simulink library "fluidDynamicSurface_cl"  (R2018b)
settings: Solver=VariableStepAuto  StartTime=0.0  StopTime=10.0  RelTol=1e-3
undefined symbols (not defined in the file or in its folder): aeroStruct
libraries: vrlib x2, vectorNormalizer_ul x2, dynamicPressure_ul x1, alphaBeta_ul x1, surfaceCoefficients_ul x1
settings Model: Creator=mcobb  LastModifiedBy=mcobb

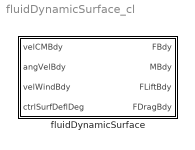
== system fluidDynamicSurface_cl ==
  fluidDynamicSurface : Subsystem  mask{aeroStruct=aeroStruct}
      mask prompts: aeroStruct "Aerodynamic surface structure"
      mask help:
      | Input must be an 1×N struct array with fields:
      |     refArea
      |     aeroCentPosVec
      |     spanUnitVec
      |     chordUnitVec
      |     fluidDensity
      |     CL
      |     CD
      |     alpha
      |     GainCL
      |     GainCD
      |
      | where N is the number of aerodynamic surfaces
      mask init:
      | fluidDynamicSurface_init

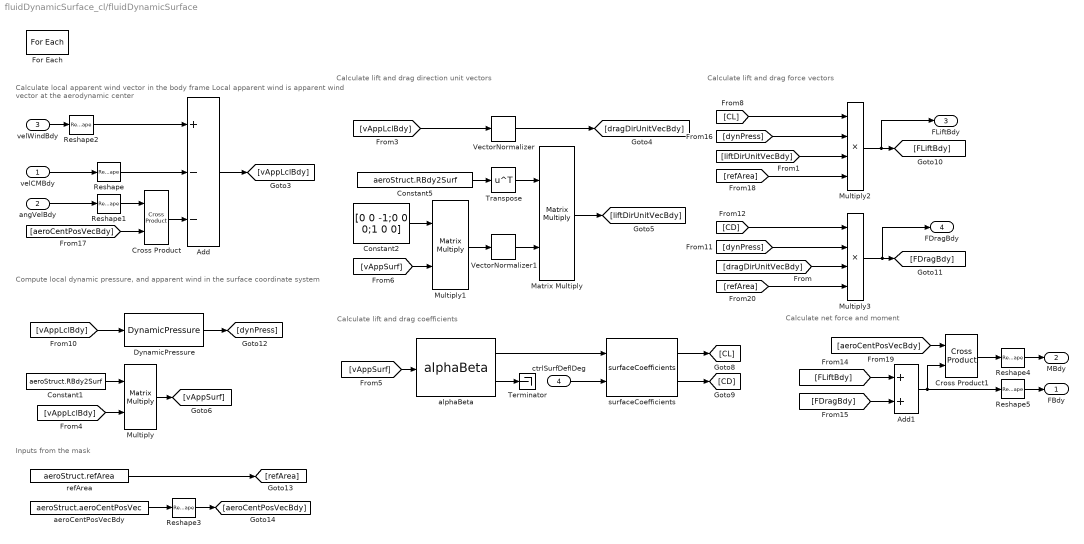
== system fluidDynamicSurface_cl/fluidDynamicSurface ==
  note: Calculate net force and moment
  note: Calculate lift and drag force vectors
  note: Calculate lift and drag coefficients
  note: Compute local dynamic pressure,
      | and apparent wind in the surface coordinate system
  note: Inputs from the mask
  note: Calculate lift and drag direction unit vectors
  note: Calculate local apparent wind vector in the body frame
      | Local apparent wind is apparent wind vector at the aerodynamic center
  velCMBdy : Inport
  angVelBdy : Inport  Port=2
  velWindBdy : Inport  Port=3
  ctrlSurfDeflDeg : Inport  Port=4  Partition=on  PartitionDimension=1  PartitionWidth=1  PartitionOffset=0
  Add : Sum  Inputs=+--
  Add1 : Sum
  Constant1 : Constant  Value=aeroStruct.RBdy2Surf
  Constant2 : Constant  Value=[0 0 -1;0 0 0;1 0 0]
  Constant5 : Constant  Value=aeroStruct.RBdy2Surf
  Cross Product : vrlib/Utilities/Cross Product
      settings: SourceProductBaseCode=VR
  Cross Product1 : vrlib/Utilities/Cross Product
      settings: SourceProductBaseCode=VR
  DynamicPressure : dynamicPressure_ul/DynamicPressure  rho=aeroStruct.fluidDensity
  For Each : ForEach  DisableCoverage=on  IterateSubsysMaskParameter=on  SubsysMaskParameterIterationDimension=2  IndexMode=One-based
  Matrix Multiply : Product  Multiplication=Matrix(*)
  Multiply : Product  Multiplication=Matrix(*)
  Multiply1 : Product  Multiplication=Matrix(*)
  Multiply2 : Product  Inputs=4
  Multiply3 : Product  Inputs=4
  Reshape{,1..5} (6 alike) : Reshape  OutputDimensionality=Column vector (2-D)
  Terminator : Terminator
  Transpose : Math  Operator=transpose  SaturateOnIntegerOverflow=on
  "VectorNormalizer " : vectorNormalizer_ul/VectorNormalizer   SystemSampleTime=-1
  VectorNormalizer1 : vectorNormalizer_ul/VectorNormalizer   SystemSampleTime=-1
  aeroCentPosVecBdy : Constant  Value=aeroStruct.aeroCentPosVec
  alphaBeta : alphaBeta_ul/alphaBeta  SystemSampleTime=-1
  refArea : Constant  Value=aeroStruct.refArea
  surfaceCoefficients : surfaceCoefficients_ul/surfaceCoefficients  SystemSampleTime=-1
  FBdy : Outport  ConcatenationDimension=2
  MBdy : Outport  Port=2  ConcatenationDimension=2
  FLiftBdy : Outport  Port=3  ConcatenationDimension=2
  FDragBdy : Outport  Port=4  ConcatenationDimension=2
  wires:
  Cross Product/1 -> Add/3
  velWindBdy/1 -> Reshape2/1
  velCMBdy/1 -> Reshape/1
  angVelBdy/1 -> Reshape1/1
  Reshape/1 -> Add/2
  Reshape2/1 -> Add/1
  Reshape1/1 -> Cross Product/1
  [aeroCentPosVecBdy] -> Cross Product/2
  Add/1 -> [vAppLclBdy]
  [vAppLclBdy] -> "VectorNormalizer "/1
  "VectorNormalizer "/1 -> [dragDirUnitVecBdy]
  Constant1/1 -> Multiply/1
  [vAppLclBdy] -> Multiply/2
  Multiply/1 -> [vAppSurf]
  [vAppSurf] -> alphaBeta/1
  [vAppSurf] -> Multiply1/2
  Constant2/1 -> Multiply1/1
  Multiply1/1 -> VectorNormalizer1/1
  alphaBeta/2 -> Terminator/1
  surfaceCoefficients/1 -> [CL]
  surfaceCoefficients/2 -> [CD]
  [CL] -> Multiply2/1
  DynamicPressure/1 -> [dynPress]
  [liftDirUnitVecBdy] -> Multiply2/3
  [vAppLclBdy] -> DynamicPressure/1
  Multiply2/1 -> FLiftBdy/1, [FLiftBdy]
  Multiply3/1 -> FDragBdy/1, [FDragBdy]
  [dragDirUnitVecBdy] -> Multiply3/3
  [dynPress] -> Multiply3/2
  [CD] -> Multiply3/1
  Add1/1 -> Reshape5/1, Cross Product1/2
  [FDragBdy] -> Add1/2
  [FLiftBdy] -> Add1/1
  Constant5/1 -> Transpose/1
  Matrix Multiply/1 -> [liftDirUnitVecBdy]
  Transpose/1 -> Matrix Multiply/1
  VectorNormalizer1/1 -> Matrix Multiply/2
  [dynPress] -> Multiply2/2
  Cross Product1/1 -> Reshape4/1
  aeroCentPosVecBdy/1 -> Reshape3/1
  [refArea] -> Multiply2/4
  [refArea] -> Multiply3/4
  [aeroCentPosVecBdy] -> Cross Product1/1
  refArea/1 -> [refArea]
  Reshape3/1 -> [aeroCentPosVecBdy]
  Reshape4/1 -> MBdy/1
  Reshape5/1 -> FBdy/1
  ctrlSurfDeflDeg/1 -> surfaceCoefficients/2
  alphaBeta/1 -> surfaceCoefficients/1
